simulink model "two_fsk"  (R2021a)
settings: Solver=VariableStepAuto  StartTime=0.0  StopTime=10.0  RelTol=1e-3
libraries: dsparch4 x4, dspsigops x2, commchan3 x1, commrandsrc3 x1, commsink2 x1
settings Model: Creator=27734  LastModifiedBy=27734

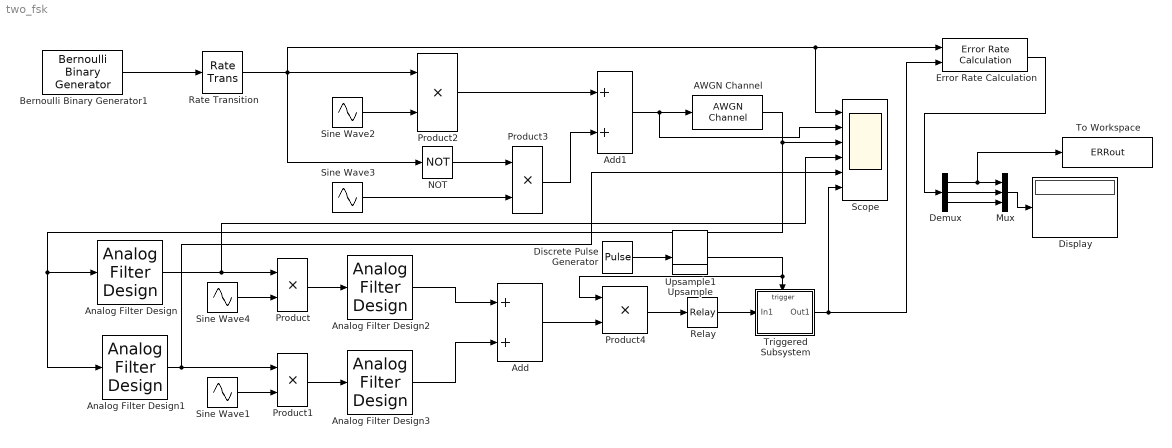
== system two_fsk ==
  AWGN Channel : commchan3/AWGN Channel  InputProcessing=Columns as channels (frame based)  seed=61  noiseMode=Variance from mask  EbNodB=10  EsNodB=10  SNRdB=10  bitsPerSym=1  Ps=1  Tsym=1  variance=0.1
  Add : Sum
  Add1 : Sum
  Analog Filter Design : dsparch4/Analog Filter Design  method=Butterworth  filttype=Bandpass  N=5  Wlo=1*2*pi  Whi=4*2*pi  Rp=2  Rs=40
  Analog Filter Design1 : dsparch4/Analog Filter Design  method=Butterworth  filttype=Bandpass  N=5  Wlo=5*2*pi  Whi=9*2*pi  Rp=2  Rs=40
  Analog Filter Design2 : dsparch4/Analog Filter Design  method=Butterworth  filttype=Lowpass  N=5  Wlo=3*2*pi  Whi=80  Rp=2  Rs=40
  Analog Filter Design3 : dsparch4/Analog Filter Design  method=Butterworth  filttype=Lowpass  N=5  Wlo=9*2*pi  Whi=80  Rp=2  Rs=40
  Bernoulli Binary Generator1 : commrandsrc3/Bernoulli Binary Generator  ProbabilityOfZero=0.5  SeedSource=Parameter  Seed=61  SampleTime=1  SamplesPerFrame=1  OutputDataType=double  SimulateUsing=Interpreted execution
  Demux : Demux  Outputs=3
  Discrete Pulse Generator : DiscretePulseGenerator  PhaseDelay=2  SampleTime=0.01
  Display : Display
  Error Rate Calculation : commsink2/Error Rate Calculation  N=0  st_delay=0  cp_mode=Entire frame  subframe=[]  PMode=Port  WsName=ErrorVec  RsMode2=off  stop=off  numErr=100  maxBits=1e6
  Mux : Mux  Inputs=3
  NOT : Logic  Operator=NOT  AllPortsSameDT=off  OutDataTypeStr=boolean
  Product{,1..4} (5 alike) : Product  RndMeth=Zero
  Rate Transition : RateTransition
  Relay : Relay
  Scope : Scope  NumInputPorts=6
  Sine Wave1 : Sin  Amplitude=2  Frequency=2*pi*8  SampleTime=0.002
  Sine Wave2 : Sin  Amplitude=2  Frequency=2*pi*2  SampleTime=0.002
  Sine Wave3 : Sin  Amplitude=2  Frequency=2*pi*8  SampleTime=0.002
  Sine Wave4 : Sin  Amplitude=2  Frequency=2*pi*2  SampleTime=0.002
  To Workspace : ToWorkspace  VariableName=ERRout  SaveFormat=Structure  SampleTime=-1
  Triggered Subsystem : Subsystem  TreatAsAtomicUnit=on
  Upsample : dspsigops/Upsample  N=5  phase=0  InputProcessing=Columns as channels (frame based)  RateOptions=Allow multirate processing  ic=0  mode=Unused parameter value
  Upsample1 : dspsigops/Upsample  N=5  phase=0  InputProcessing=Columns as channels (frame based)  RateOptions=Allow multirate processing  ic=0  mode=Unused parameter value
  wires:
  Demux/2 -> Mux/2
  Demux/3 -> Mux/3
  Mux/1 -> Display/1
  Demux/1 -> To Workspace/1, Mux/1
  Sine Wave4/1 -> Product/2
  Analog Filter Design1/1 -> Scope/5, Product1/1
  Sine Wave1/1 -> Product1/2
  Product/1 -> Analog Filter Design2/1
  Product1/1 -> Analog Filter Design3/1
  Analog Filter Design2/1 -> Add/1
  Analog Filter Design3/1 -> Add/2
  Add/1 -> Product4/2
  Product4/1 -> Relay/1
  Relay/1 -> Triggered Subsystem/1(In1)
  Bernoulli Binary Generator1/1 -> Rate Transition/1
  Sine Wave2/1 -> Product2/2
  Sine Wave3/1 -> Product3/2
  NOT/1 -> Product3/1
  Product2/1 -> Add1/1
  Product3/1 -> Add1/2
  Discrete Pulse Generator/1 -> Upsample/1
  Upsample/1 -> Product4/1, Triggered Subsystem/Trigger
  Add1/1 -> Scope/2, AWGN Channel/1
  Rate Transition/1 -> Scope/1, Error Rate Calculation/1, Product2/1, NOT/1
  AWGN Channel/1 -> Analog Filter Design/1, Analog Filter Design1/1, Scope/3
  Triggered Subsystem/1(Out1) -> Scope/6, Error Rate Calculation/2
  Error Rate Calculation/1 -> Demux/1
  Analog Filter Design/1 -> Scope/4, Product/1

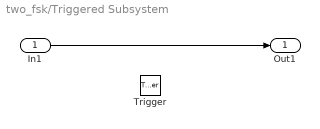
== system two_fsk/Triggered Subsystem ==
  In1 : Inport
  Trigger : TriggerPort  VariantControl=(inherit)
  Out1 : Outport
  wires:
  In1/1 -> Out1/1
